simulink model "FilterFramework"  (R2023b)
settings: Solver=FixedStepDiscrete  StartTime=0.0  StopTime=0.2  RelTol=1e-3
values from neighbouring files (symbols this model uses):
  a = [1, -2.1485451, 2.2390905, -1.1509858, 0.2532257]    [Lab_One.m]
  b = [0.0355267, 0.0306650, 0.0581951, 0.0306650, 0.0355267]    [Lab_One.m]
  fs = 16e3    (= 16000)    [Lab_One.m]
libraries: dspsrcs4 x2
settings Model: Creator=rdanse  LastModifiedBy=elfo
settings SolverCC: AlgebraicLoopSolver=TrustRegion  AutoInsertRateTranBlk=on
settings DataIOCC: LimitDataPoints=on  SaveOutput=off  SignalLogging=off  SaveTime=off
settings OptimizationCC: LifeSpan=inf  SimCompilerOptimization=on
settings DebuggingCC: AlgebraicLoopMsg=error  SingleTaskRateTransMsg=error  UnconnectedInputMsg=warning  UnconnectedOutputMsg=warning  UnconnectedLineMsg=warning  AllowSymbolicDim=off  SFUnexpectedBacktrackingDiag=warning  SFNoUnconditionalDefaultTransitionDiag=warning  SFExecutionAtInitializationDiag=none  ArithmeticOperatorsInVariantConditions=warning
settings ModelReferenceCC: EnableRefExpFcnMdlSchedulingChecks=on
settings SFSimCC: SimUseLocalCustomCode=off  CustomCodeUndefinedFunction=UseInterfaceOnly
settings RTWCC: RTWUseLocalCustomCode=off
settings CodeAppCC: StateflowObjectComments=on
settings GRTTargetCC: TargetLangStandard=C89/C90 (ANSI)
settings ConfigComp: CovMetricSettings=dw  CovSaveCumulativeToWorkspaceVar=on  CovSaveSingleToWorkspaceVar=on  CovExternalEMLEnable=off  CovSFcnEnable=off

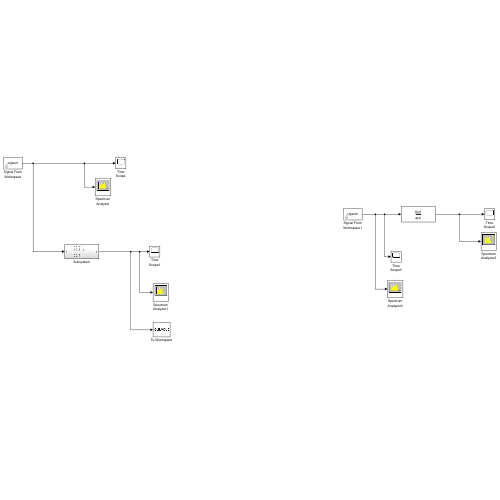
[thumbnail: Simulink's stored preview of the top-level diagram]
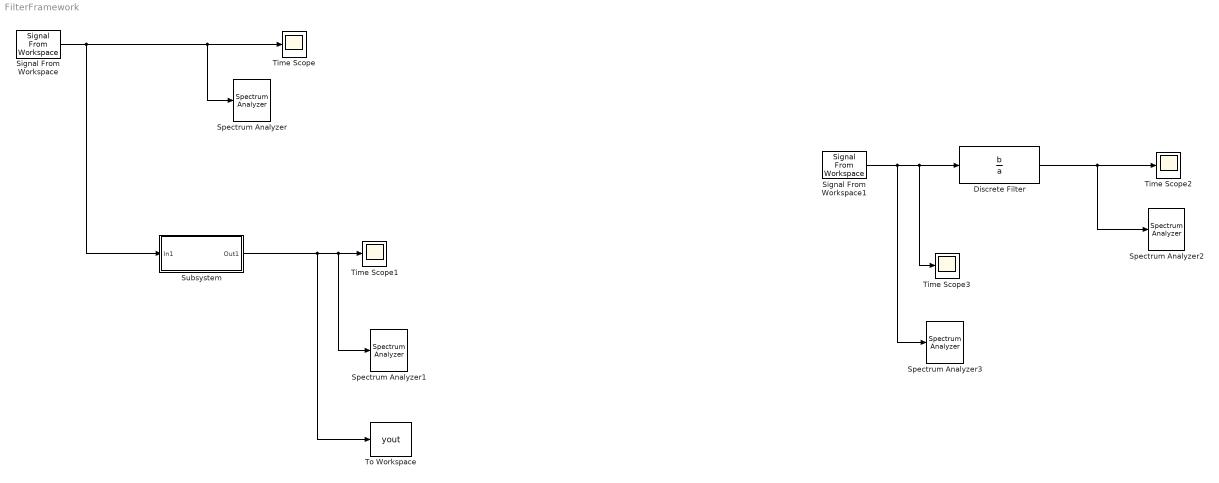
== system FilterFramework ==
  Discrete Filter : DiscreteFilter  Numerator=b  Denominator=a  InputProcessing=Columns as channels (frame based)  FilterStructure=Direct form II transposed  a0EqualsOne=on
  Signal From Workspace : dspsrcs4/Signal From Workspace  X=sigsum  Ts=1/fs  nsamps=1  OutputAfterFinalValue=Cyclic repetition  ignoreOrWarnInputAndFrameLengths=off  OutputFrames=off
  Signal From Workspace1 : dspsrcs4/Signal From Workspace  X=sigsum  Ts=1/fs  nsamps=1  OutputAfterFinalValue=Cyclic repetition  ignoreOrWarnInputAndFrameLengths=off  OutputFrames=off
  Spectrum Analyzer : SpectrumAnalyzer  WindowPosition=[1485.000000,248.000000,1145.000000,792.000000,]  ScopeFrameLocation=window  SpectrumType=Power density  SpectrumUnits=dBm/Hz  YLimits=[-149.99904309,-42.95173174]  ColorLimits=[-80 20]
  Spectrum Analyzer1 : SpectrumAnalyzer  WindowPosition=[1026.000000,502.000000,858.000000,588.000000,]  ScopeFrameLocation=window  SpectrumType=Power density  SpectrumUnits=dBm/Hz  YLimits=[-220.48413424,-35.22615224]  ColorLimits=[-80 20]
  Spectrum Analyzer2 : SpectrumAnalyzer  WindowPosition=[854.000000,553.000000,800.000000,500.000000,]  ScopeFrameLocation=window  SpectrumType=Power density  SpectrumUnits=dBm/Hz  YLimits=[-213.92033927,-42.64464736]  ColorLimits=[-80 20]
  Spectrum Analyzer3 : SpectrumAnalyzer  WindowPosition=[2357.000000,290.000000,800.000000,500.000000,]  ScopeFrameLocation=window  SpectrumType=Power density  SpectrumUnits=dBm/Hz  YLimits=[-152.65022863,-49.34631593]  ColorLimits=[-80 20]
  Subsystem : Subsystem
  Time Scope{,1..3} (4 alike) : Scope
  To Workspace : ToWorkspace  VariableName=yout  SampleTime=-1
      settings: Save2DSignal=2-D array (concatenate along first dimension)
  wires:
  Signal From Workspace/1 -> Subsystem/1(In1), Spectrum Analyzer/1, Time Scope/1
  Subsystem/1(Out1) -> To Workspace/1, Spectrum Analyzer1/1, Time Scope1/1
  Signal From Workspace1/1 -> Spectrum Analyzer3/1, Time Scope3/1, Discrete Filter/1
  Discrete Filter/1 -> Spectrum Analyzer2/1, Time Scope2/1

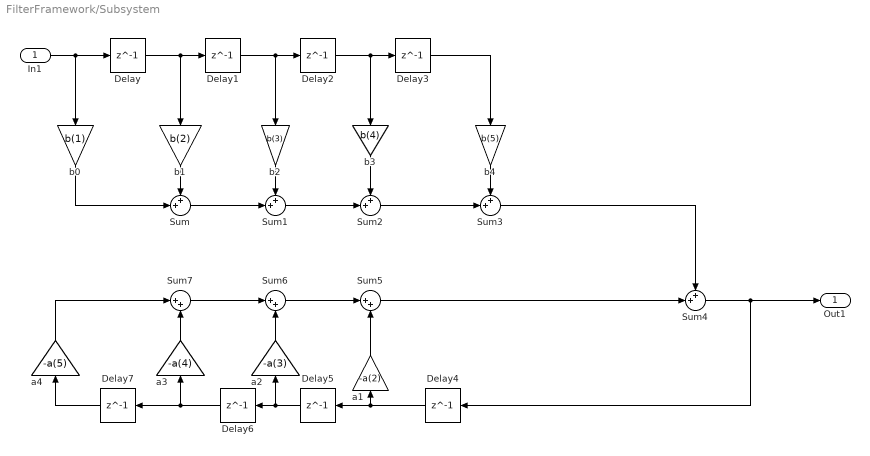
== system FilterFramework/Subsystem ==
  In1 : Inport
  Delay{,1..7} (8 alike) : Delay  DelayLength=1
  Sum{,1..4} (5 alike) : Sum  Inputs=++|
  Sum5 : Sum  Inputs=|++
  Sum6 : Sum  Inputs=|++
  Sum7 : Sum  Inputs=|++
  a1 : Gain  Gain=-a(2)
  a2 : Gain  Gain=-a(3)
  a3 : Gain  Gain=-a(4)
  a4 : Gain  Gain=-a(5)
  b0 : Gain  Gain=b(1)
  b1 : Gain  Gain=b(2)
  b2 : Gain  Gain=b(3)
  b3 : Gain  Gain=b(4)
  b4 : Gain  Gain=b(5)
  Out1 : Outport
  wires:
  In1/1 -> b0/1, Delay/1
  Delay/1 -> b1/1, Delay1/1
  Delay1/1 -> Delay2/1, b2/1
  Delay2/1 -> b3/1, Delay3/1
  Delay3/1 -> b4/1
  b0/1 -> Sum/2
  b1/1 -> Sum/1
  Sum/1 -> Sum1/2
  Sum1/1 -> Sum2/2
  Sum2/1 -> Sum3/2
  b4/1 -> Sum3/1
  Sum3/1 -> Sum4/1
  Sum4/1 -> Delay4/1, Out1/1
  Sum5/1 -> Sum4/2
  Sum6/1 -> Sum5/1
  Sum7/1 -> Sum6/1
  a4/1 -> Sum7/1
  a3/1 -> Sum7/2
  a2/1 -> Sum6/2
  a1/1 -> Sum5/2
  Delay4/1 -> Delay5/1, a1/1
  Delay5/1 -> a2/1, Delay6/1
  Delay6/1 -> a3/1, Delay7/1
  Delay7/1 -> a4/1
  b2/1 -> Sum1/1
  b3/1 -> Sum2/1
